simulink library "can_lib"  (Simulink 7.0)
undefined symbols (not defined in the file): CAN_DEVICE_A, UNDEFINED_VALUE
settings Model: Creator=WX  LastModifiedBy=WX

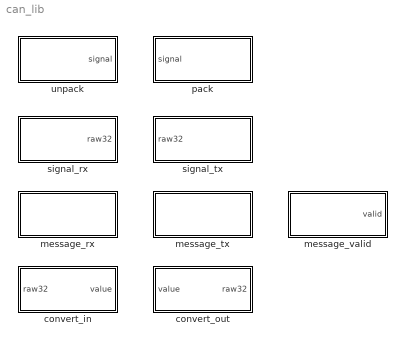
== system can_lib ==
  convert_in : Subsystem  mask(ConvertIn){gain=UNDEFINED_VALUE, offset=UNDEFINED_VALUE}
      mask help:
      | Conversion Formula
      |
      | The conversion formula is
      |
      | raw_value = (physical_value - Offset) / Factor
      |
      | where physical_value is the value of the signal after it is saturated using the specified Min and Max values. raw_value is the packed signal value.
  convert_out : Subsystem  mask(ConvertOut){gain=UNDEFINED_VALUE, offset=UNDEFINED_VALUE}
      mask help:
      | Conversion Formula
      |
      | The conversion formula is
      |
      | raw_value = (physical_value - Offset) / Factor
      |
      | where physical_value is the value of the signal after it is saturated using the specified Min and Max values. raw_value is the packed signal value.
  message_rx : Subsystem  TreatAsAtomicUnit=on  mask{dev=CAN_DEVICE_A, id=0}
      mask prompts: dev "CAN Device:"; id "CAN ID"
      mask Display: fprintf('ID: 0x%08X', id);
  message_tx : Subsystem  TreatAsAtomicUnit=on  mask{dev=CAN_DEVICE_A, id=0}
      mask prompts: dev "CAN Device:"; id "CAN ID"
      mask Display: fprintf('ID: 0x%08X', id);
  message_valid : Subsystem  mask{dev=CAN_DEVICE_A, id=0}
      mask prompts: dev "CAN Device:"; id "CAN ID"
      mask Display: fprintf('device %d valid\nID: 0x%08X', dev, id);
  pack : Subsystem  TreatAsAtomicUnit=on  mask(CAN_Pack){dbc_file=}
      mask prompts: dbc_file "CANdb File"
      settings: OpenFcn=can_pack
  signal_rx : Subsystem  TreatAsAtomicUnit=on  mask{dev=CAN_DEVICE_A, id=0, bit_start=0, bit_len=0}
      mask prompts: dev "CAN Device:"; id "CAN ID"; bit_start "Bit Start"; bit_len "Bit Length"
  signal_tx : Subsystem  TreatAsAtomicUnit=on  mask{dev=CAN_DEVICE_A, id=0, bit_start=0, bit_len=0}
      mask prompts: dev "CAN Device:"; id "CAN ID"; bit_start "Bit Start"; bit_len "Bit Length"
  unpack : Subsystem  TreatAsAtomicUnit=on  mask(CAN_Unpack){dbc_file=}
      mask prompts: dbc_file "CANdb File"
      mask init:
      | dbc_file='';
      settings: OpenFcn=can_unpack

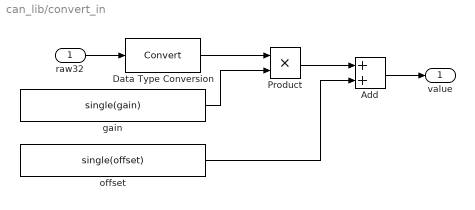
== system can_lib/convert_in ==
  raw32 : Inport  OutDataType=sfix(16)  OutScaling=2^0
  Add : Sum  OutDataType=sfix(16)  OutScaling=2^-10
  Data Type Conversion : DataTypeConversion  OutDataTypeMode=single  OutDataType=sfix(16)  OutScaling=2^0
  Product : Product  OutDataType=sfix(16)  OutScaling=2^0  RndMeth=Zero
  gain : Constant  Value=single(gain)  OutDataTypeMode=single  OutDataType=sfix(16)  OutScaling=2^0
  offset : Constant  Value=single(offset)  OutDataTypeMode=single  OutDataType=sfix(16)  OutScaling=2^0
  value : Outport  OutDataType=sfix(16)  OutScaling=2^0
  wires:
  raw32/1 -> Data Type Conversion/1
  gain/1 -> Product/2
  Product/1 -> Add/1
  offset/1 -> Add/2
  Add/1 -> value/1
  Data Type Conversion/1 -> Product/1

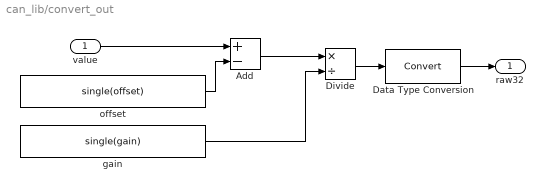
== system can_lib/convert_out ==
  value : Inport  OutDataType=sfix(16)  OutScaling=2^0
  Add : Sum  Inputs=+-  OutDataType=sfix(16)  OutScaling=2^-10
  Data Type Conversion : DataTypeConversion  OutDataTypeMode=uint32  OutDataType=sfix(16)  OutScaling=2^0  RndMeth=Nearest
  Divide : Product  Inputs=*/  OutDataType=sfix(16)  OutScaling=2^-10
  gain : Constant  Value=single(gain)  OutDataTypeMode=single  OutDataType=sfix(16)  OutScaling=2^0
  offset : Constant  Value=single(offset)  OutDataTypeMode=single  OutDataType=sfix(16)  OutScaling=2^0
  raw32 : Outport  OutDataType=sfix(16)  OutScaling=2^0
  wires:
  value/1 -> Add/1
  offset/1 -> Add/2
  Divide/1 -> Data Type Conversion/1
  Add/1 -> Divide/1
  gain/1 -> Divide/2
  Data Type Conversion/1 -> raw32/1

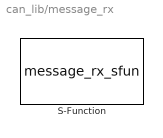
== system can_lib/message_rx ==
  S-Function : S-Function  FunctionName=message_rx_sfun  Parameters=uint8(dev),uint32(id),

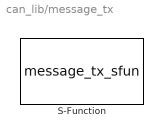
== system can_lib/message_tx ==
  S-Function : S-Function  FunctionName=message_tx_sfun  Parameters=uint8(dev),uint32(id)

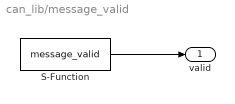
== system can_lib/message_valid ==
  S-Function : S-Function  FunctionName=message_valid  Parameters=uint8(dev),uint32(id)
  valid : Outport  OutDataType=fixdt(1, 16)  OutScaling=2^0
  wires:
  S-Function/1 -> valid/1

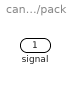
== system can_lib/pack ==
  signal : Inport  OutDataType=fixdt(1, 16)  OutScaling=2^0

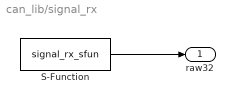
== system can_lib/signal_rx ==
  S-Function : S-Function  FunctionName=signal_rx_sfun  Parameters=uint8(dev),uint32(id),uint8(bit_start),uint8(bit_len)
  raw32 : Outport  OutDataType=fixdt(1, 16)  OutScaling=2^0
  wires:
  S-Function/1 -> raw32/1

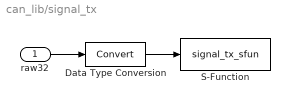
== system can_lib/signal_tx ==
  raw32 : Inport  OutDataType=fixdt(1, 16)  OutScaling=2^0
  Data Type Conversion : DataTypeConversion  OutDataTypeMode=uint32  OutDataType=sfix(16)  OutScaling=2^0
  S-Function : S-Function  FunctionName=signal_tx_sfun  Parameters=uint8(dev),uint32(id),uint8(bit_start),uint8(bit_len)
  wires:
  raw32/1 -> Data Type Conversion/1
  Data Type Conversion/1 -> S-Function/1

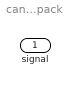
== system can_lib/unpack ==
  signal : Outport  OutDataType=fixdt(1, 16)  OutScaling=2^0
